simulink model "rlpitch"  (R2019b)
settings: Solver=ode45  StartTime=0.0  StopTime=50  RelTol=1e-3  EnableMultiTasking=on
undefined symbols (not defined in the file or in its folder): DiscIntNeverNeededParam, Ts
libraries: simulink x3, rllib x1
settings Model: Creator=The MathWorks, Inc.  LastModifiedBy=Adyasha
settings DataIOCC: LimitDataPoints=on  SaveFormat=Array  ReturnWorkspaceOutputs=off  SignalLoggingName=logsOut
settings OptimizationCC: ExpressionDepthLimit=2147483647  InitFltsAndDblsToZero=on  LifeSpan=inf
settings DebuggingCC: SaveWithParameterizedLinksMsg=none  UnderspecifiedInitializationDetection=Classic  MergeDetectMultiDrivingBlocksExec=none  SignalResolutionControl=TryResolveAllWithWarning  MultiTaskDSMMsg=warning  FcnCallInpInsideContextMsg=warning  AllowSymbolicDim=off  StateNameClashWarn=warning  SFUnexpectedBacktrackingDiag=warning  SFNoUnconditionalDefaultTransitionDiag=warning  SFExecutionAtInitializationDiag=none  ArithmeticOperatorsInVariantConditions=warning
settings HardwareCC: ProdBitPerPointer=32  ProdBitPerSizeT=32  ProdBitPerPtrDiffT=32  ProdLargestAtomicFloat=None  ProdIntDivRoundTo=Undefined  ProdEndianess=Unspecified  ProdWordSize=32  ProdHWDeviceType=Specified
settings ModelReferenceCC: PropagateSignalLabelsOutOfModel=off
settings SFSimCC: SimUseLocalCustomCode=off  CustomCodeUndefinedFunction=UseInterfaceOnly
settings RTWCC: RTWUseLocalCustomCode=off
settings CodeAppCC: StateflowObjectComments=on
settings GRTTargetCC: TargetFcnLib=ansi_tfl_tmw.mat  TargetLangStandard=C89/C90 (ANSI)  GeneratePreprocessorConditionals=Disable all  CombineOutputUpdateFcns=off  GRTInterface=on
settings ConfigComp: CovMetricSettings=dw  CovHtmlReporting=on  CovSaveCumulativeToWorkspaceVar=on  CovSaveSingleToWorkspaceVar=on  CovExternalEMLEnable=off

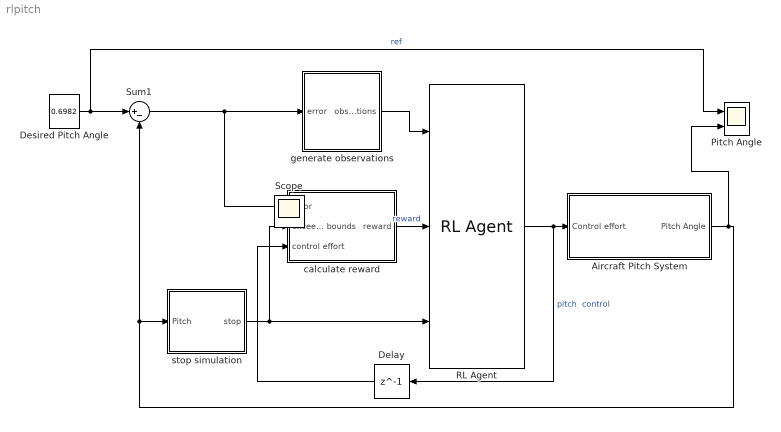
== system rlpitch ==
  Aircraft Pitch System : Subsystem
  Delay : Delay  DelayLength=1  InitialCondition=0
  Desired Pitch Angle : Constant  Value=0.6982
  Pitch Angle : Scope  NumInputPorts=2
  RL Agent : rllib/RL Agent  Agent=agent  ProvideReward=on  ProvideIsDone=on  ProvideCumRwd=off  TreatAsDirectFeedthrough=on  CollectLoggedSignals=on  CollectModelStates=on
      settings: SourceProductName=Reinforcement Learning Toolbox
  Sum1 : Sum  Inputs=|+-  SaturateOnIntegerOverflow=on
  calculate reward : Subsystem
  generate observations : Subsystem
  stop simulation : Subsystem
  Scope : Scope
  wires:
  Desired Pitch Angle/1 -> Pitch Angle/1, Sum1/1  "ref"
  Sum1/1 -> calculate reward/1(error), generate observations/1(error)
  stop simulation/1(stop) -> RL Agent/3, calculate reward/2(exceeds bounds)
  calculate reward/1(reward) -> RL Agent/2  "reward"
  generate observations/1(observations) -> RL Agent/1
  Aircraft Pitch System/1(Pitch Angle) -> Pitch Angle/2, Sum1/2, stop simulation/1(Pitch)
  RL Agent/1 -> Delay/1, Aircraft Pitch System/1(Control effort)  "pitch  control"
  Delay/1 -> calculate reward/3(control effort)

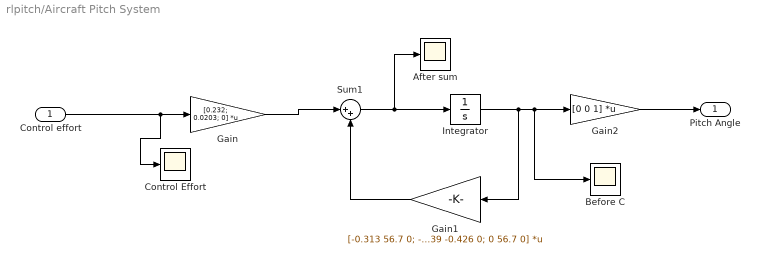
== system rlpitch/Aircraft Pitch System ==
  Control effort : Inport
  After sum : Scope
  Before C : Scope
  Control Effort : Scope
  Gain : Gain  Gain=[0.232; 0.0203; 0]  Multiplication=Matrix(K*u)
  Gain1 : Gain  Gain=[-0.313 56.7 0; -0.0139 -0.426 0; 0 56.7 0]  Multiplication=Matrix(K*u)
  Gain2 : Gain  Gain=[0 0 1]  Multiplication=Matrix(K*u)
  Integrator : Integrator
  Sum1 : Sum  Inputs=|++
  Pitch Angle : Outport  VectorParamsAs1DForOutWhenUnconnected=off
  wires:
  Gain/1 -> Sum1/1
  Sum1/1 -> After sum/1, Integrator/1
  Integrator/1 -> Gain1/1, Before C/1, Gain2/1
  Gain1/1 -> Sum1/2
  Control effort/1 -> Gain/1, Control Effort/1
  Gain2/1 -> Pitch Angle/1

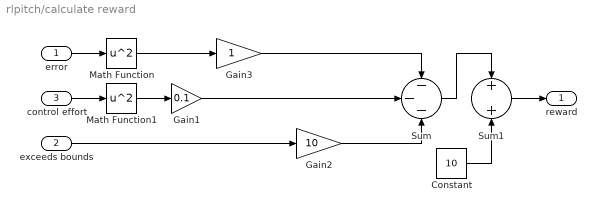
== system rlpitch/calculate reward ==
  error : Inport
  exceeds bounds : Inport  Port=2
  control effort : Inport  Port=3
  Constant : Constant  Value=10
  Gain1 : Gain  Gain=0.1
  Gain2 : Gain  Gain=10
  Gain3 : Gain
  Math Function : Math  Operator=square  SignedPower=off  SaturateOnIntegerOverflow=on
  Math Function1 : Math  Operator=square  SignedPower=off  SaturateOnIntegerOverflow=on
  Sum : Sum  Inputs=---  OutDataTypeStr=double
  Sum1 : Sum  OutDataTypeStr=double
  reward : Outport  VectorParamsAs1DForOutWhenUnconnected=off
  wires:
  Gain2/1 -> Sum/3
  exceeds bounds/1 -> Gain2/1
  error/1 -> Math Function/1
  control effort/1 -> Math Function1/1
  Math Function1/1 -> Gain1/1
  Gain1/1 -> Sum/2
  Math Function/1 -> Gain3/1
  Gain3/1 -> Sum/1
  Sum/1 -> Sum1/1
  Sum1/1 -> reward/1
  Constant/1 -> Sum1/2

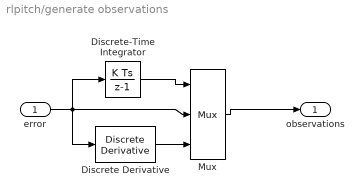
== system rlpitch/generate observations ==
  error : Inport
  Discrete Derivative : simulink/Discrete/Discrete Derivative  gainval=1.0  ICPrevScaledInput=0.0  OutMin=[]  OutMax=[]  OutDataType=fixdt(1, 16)  OutScaling=2^-10  DoSatur=off
  Discrete-Time Integrator : DiscreteIntegrator  SampleTime=Ts  ICPrevOutput=DiscIntNeverNeededParam  ICPrevScaledInput=DiscIntNeverNeededParam
  Mux : Mux  Inputs=3
  observations : Outport  VectorParamsAs1DForOutWhenUnconnected=off
  wires:
  Discrete-Time Integrator/1 -> Mux/1
  error/1 -> Mux/2, Discrete Derivative/1, Discrete-Time Integrator/1
  Mux/1 -> observations/1
  Discrete Derivative/1 -> Mux/3

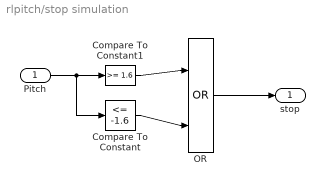
== system rlpitch/stop simulation ==
  Pitch : Inport
  Compare To Constant : simulink/Logic and Bit Operations/Compare To Constant  relop=<=  const=-1.6  OutDataTypeStr=boolean
  Compare To Constant1 : simulink/Logic and Bit Operations/Compare To Constant  relop=>=  const=1.6  OutDataTypeStr=boolean
  OR : Logic  Operator=OR  IconShape=distinctive  AllPortsSameDT=off  OutDataTypeStr=boolean
  stop : Outport  VectorParamsAs1DForOutWhenUnconnected=off
  wires:
  Pitch/1 -> Compare To Constant/1, Compare To Constant1/1
  Compare To Constant/1 -> OR/2
  Compare To Constant1/1 -> OR/1
  OR/1 -> stop/1
